simulink model "speed_planning"  (R2021a)
settings: Solver=FixedStepAuto  StartTime=0.0  StopTime=15  FixedStep=0.002  RelTol=1e-3
InitFcn:
  | clc;clear all;
  | ego_velocity_init = 10.0;
  | obstacle_velocity_init = 20.0;
  | obstacle_distance_init = 50.0;
  | obstacle_accelaration_init = -3.0;
  | 
  | wn = 5.0;
  | zeta = 0.85;
StopFcn:
  | PlotResult
  | figure
  | SecondOrderSystemRespond(wn, zeta)
libraries: simulink x1
settings Model: Creator=mpt  LastModifiedBy=mapen
settings SolverCC: AlgebraicLoopSolver=TrustRegion
settings DebuggingCC: SFMachineParentedDataDiag=warning

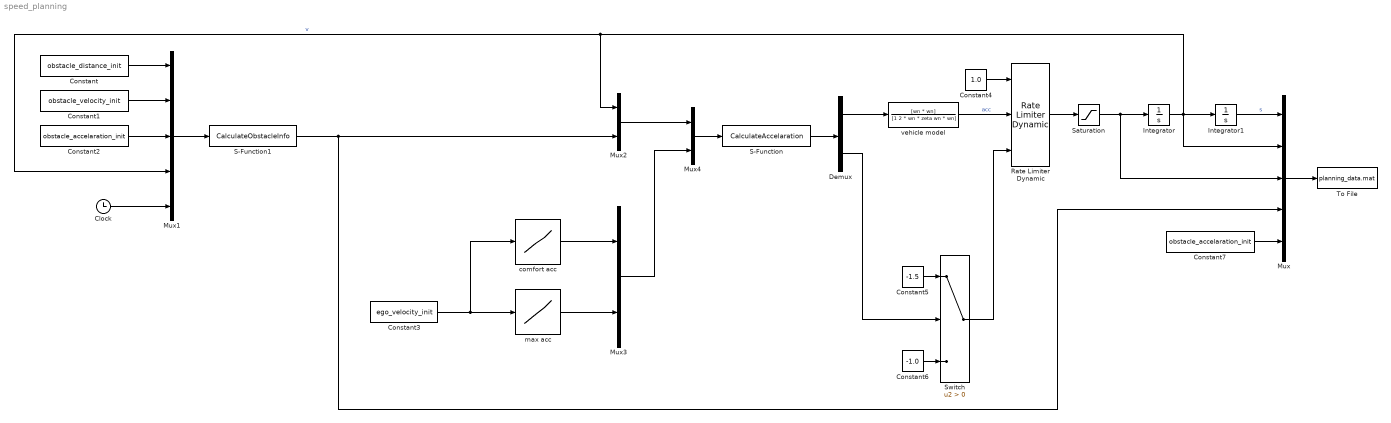
== system speed_planning ==
  Clock : Clock
  Constant : Constant  Value=obstacle_distance_init
  Constant1 : Constant  Value=obstacle_velocity_init
  Constant2 : Constant  Value=obstacle_accelaration_init
  Constant3 : Constant  Value=ego_velocity_init
  Constant4 : Constant  Value=1.0
  Constant5 : Constant  Value=-1.5
  Constant6 : Constant  Value=-1.0
  Constant7 : Constant  Value=obstacle_accelaration_init
  Demux : Demux  Outputs=2
  Integrator : Integrator  InitialCondition=ego_velocity_init  LimitOutput=on  UpperSaturationLimit=150 / 3.6  LowerSaturationLimit=0
  Integrator1 : Integrator  LimitOutput=on  LowerSaturationLimit=0
  Mux : Mux  Inputs=5
  Mux1 : Mux  Inputs=5
  Mux2 : Mux  Inputs=2
  Mux3 : Mux  Inputs=2
  Mux4 : Mux  Inputs=2
  Rate Limiter Dynamic : simulink/Discontinuities/Rate Limiter Dynamic
  S-Function : S-Function  FunctionName=CalculateAccelaration  SFunctionDeploymentMode=off  EnableBusSupport=off
  S-Function1 : S-Function  FunctionName=CalculateObstacleInfo  SFunctionDeploymentMode=off  EnableBusSupport=off
  Saturation : Saturate  UpperLimit=3.0  LowerLimit=-5.0  LinearizeAsGain=off
  Switch : Switch  Criteria=u2 > Threshold
  To File : ToFile  Filename=planning_data.mat  MatrixName=planning_data  SaveFormat=Timeseries
  comfort acc : Lookup_n-D  NumberOfTableDimensions=1  BreakpointsForDimension1=[5.0, 15.0]  Table=[-2.0, -1.0]  InternalRulePriority=Speed  RndMeth=Simplest  InputSameDT=on
  max acc : Lookup_n-D  NumberOfTableDimensions=1  BreakpointsForDimension1=[5.0, 15.0]  Table=[-3.5, -2.0]  InternalRulePriority=Speed  RndMeth=Simplest  InputSameDT=on
  vehicle model : TransferFcn  Numerator=[wn * wn]  Denominator=[1 2 * wn * zeta wn * wn]
  wires:
  Integrator/1 -> Integrator1/1, Mux/2, Mux2/1, Mux1/4  "v"
  Integrator1/1 -> Mux/1  "s"
  Mux/1 -> To File/1
  Constant/1 -> Mux1/1
  Constant1/1 -> Mux1/2
  Constant2/1 -> Mux1/3
  S-Function1/1 -> Mux/4, Mux2/2
  Constant3/1 -> comfort acc/1, max acc/1
  comfort acc/1 -> Mux3/1
  max acc/1 -> Mux3/2
  Mux4/1 -> S-Function/1
  Mux2/1 -> Mux4/1
  Mux3/1 -> Mux4/2
  Saturation/1 -> Integrator/1, Mux/3
  S-Function/1 -> Demux/1
  Demux/1 -> vehicle model/1
  vehicle model/1 -> Rate Limiter Dynamic/2  "acc"
  Rate Limiter Dynamic/1 -> Saturation/1
  Constant4/1 -> Rate Limiter Dynamic/1
  Switch/1 -> Rate Limiter Dynamic/3
  Constant5/1 -> Switch/1
  Constant6/1 -> Switch/3
  Constant7/1 -> Mux/5
  Mux1/1 -> S-Function1/1
  Clock/1 -> Mux1/5
  Demux/2 -> Switch/2
